simulink model "atrias_boom_nmStand_fullCtrl"  (R2015a)
settings: Solver=ode23t  StartTime=0.0  StopTime=t_end  FixedStep=0.001  MaxStep=1e-3  RelTol=1e-3
InitFcn:
  | addpath('../common/')
  | colors
StartFcn:
  | tic
StopFcn:
  | %stopscript
values from neighbouring files (symbols this model uses):
  A1_notch_f1 = -2*cos(fnotch_f1*sample_time)    [set_control_params.m]
  A2_notch_f1 = 1    [set_control_params.m]
  A_lpf_dtau = 1 + B1_lpf_dtau + B2_lpf_dtau    [set_control_params.m]
  ankle_stiffness = 1/2*pi    (= 1.57079632679)    [mechanical_params.m]
  B1_lpf_dtau = -2*exp(-lpf_damping*fcut_dtau*sample_time)*cos(fcut_dtau*sample_time*sqrt(1-lpf_damping^2))    [set_control_params.m]
  B1_notch_f1 = -2*exp(-notch_damping*fnotch_f1*sample_time)*cos(fnotch_f1*sample_time*sqrt(1-notch_damping^2))    [set_control_params.m]
  B2_lpf_dtau = exp(-2*lpf_damping*fcut_dtau*sample_time)    [set_control_params.m]
  B2_notch_f1 = exp(-2*notch_damping*fnotch_f1*sample_time)    [set_control_params.m]
  b_hmotor = 0    [mechanical_params.m]
  b_leg_spring = 0.075*sqrt(k_leg_spring*0.5*.25^2)    [mechanical_params.m]
  b_rotor = 0*60/(2*pi)*9.725e-5    (= 0)    [mechanical_params.m]
  boom_mount_to_center_diagonal = boom_mount_to_center / cos(pitch_mount_angle)    [mechanical_params.m]    (also in set_control_params.m)
  breakaway_friction = [25 25 25 25]    [mechanical_params.m]
  contactThr = 0.35    [set_control_params.m]
  coulomb_friction = [20 20 20 20]    [mechanical_params.m]
  d_com = (d_hip_com_to_torso_com*m_torso)/(m_torso + num_legs*m_hshaft)    [mechanical_params.m]
  delta_phi_max = 160*pi/180    (= 2.79252680319)    [mechanical_params.m]    (also in set_control_params.m)
  delta_phi_max_buffer = 20*pi/180    (= 0.349065850399)    [set_control_params.m]
  delta_phi_max_dropoff = 2*pi/180    (= 0.0349065850399)    [set_control_params.m]
  delta_phi_min = 25.5*pi/180    (= 0.445058959259)    [mechanical_params.m]    (also in set_control_params.m)
  friction_linear_zone = [0.5 0.5 0.5 0.5].*pi/180    [mechanical_params.m]
  g = 9.803    [mechanical_params.m]    (also in set_control_params.m = 9.81)
  gain_nodes_sea_torque = [0,65,350,700]    [set_control_params.m]
  HIP_MTR_MAX_CONT_TORQUE = HIP_MTR_MAX_CONT_CURRENT*HIP_MOTOR_CONSTANT*HIP_MTR_GEAR_RATIO    (= 86.0016)    [set_control_params.m]
  HIP_MTR_MAX_TORQUE = max_current_hip*Kt_hip*N_h    (= 629.28)    [mechanical_params.m]
  initial_boom_pitch = 0    [mechanical_params.m]
  initial_boom_roll = asin((initial_com_height + boom_mount_to_com + boom_mount_to_center*tan(pitch_mount_angle) - (base_12(2) + yshaft_12(2))) / (l_boom + boom_mount_to_center_diagonal))    [mechanical_params.m]
  initial_boom_yaw = 0    [mechanical_params.m]
  initial_hip_roll = 0*pi/180    (= 0)    [mechanical_params.m]
  initial_winch_angle = -12 * pi/180    (= -0.209439510239)    [mechanical_params.m]
  k_gn = m_total*g/0.01    (= 57041.421916)    [mechanical_params.m]
  k_gt = m_total*g/0.1    (= 5704.1421916)    [mechanical_params.m]
  k_leg_spring = 4118.3    [mechanical_params.m]    (also in set_control_params.m)
  K_notch_f1 = (1+B1_notch_f1+B2_notch_f1)/(1+A1_notch_f1+A2_notch_f1)    [set_control_params.m]
  k_phi = 5000    [mechanical_params.m]
  k_sea = [4118.3 4118.3 4118.3 4118.3]    [set_control_params.m]
  Kb_leg = 0.121    [mechanical_params.m]
  kd_boom_roll_Ctrl = 0    [main_1_nmStand.m]    (also in main_2_nmStand_moveBoom.m)
  kd_lateral = 2*sqrt(kp_lateral*0.8)    [set_control_params.m]
  kd_shin_max = kd_pd_avoid_limits    (= 1000)    [set_control_params.m]
  kd_shin_min = kd_pd_avoid_limits    (= 1000)    [set_control_params.m]
  kd_splay_max = kd_pd_avoid_limits    (= 1000)    [set_control_params.m]
  kd_splay_min = kd_pd_avoid_limits    (= 1000)    [set_control_params.m]
  kd_thigh_max = kd_pd_avoid_limits    (= 1000)    [set_control_params.m]
  kd_thigh_min = kd_pd_avoid_limits    (= 1000)    [set_control_params.m]
  kd_winch = td_winch*kp_winch    (= 989.239577798)    [mechanical_params.m]
  kp_boom_roll_Ctrl = 0    [main_1_nmStand.m]    (also in main_2_nmStand_moveBoom.m)
  kp_lateral = 1000    [set_control_params.m]
  kp_sea_torque = [0.3, 0.3, 6.0, 6.0]    [set_control_params.m]
  kp_shin_max = kp_pd_avoid_limits    (= 5000)    [set_control_params.m]
  kp_shin_min = kp_pd_avoid_limits    (= 5000)    [set_control_params.m]
  kp_splay_max = kp_pd_avoid_limits    (= 5000)    [set_control_params.m]
  kp_splay_min = kp_pd_avoid_limits/10    (= 500)    [set_control_params.m]
  kp_thigh_max = kp_pd_avoid_limits    (= 5000)    [set_control_params.m]
  kp_thigh_min = kp_pd_avoid_limits    (= 5000)    [set_control_params.m]
  kp_winch = winch_gravity_comp/(3*pi/180)    (= 19784.791556)    [mechanical_params.m]
  Kt_leg = 0.121    [mechanical_params.m]
  l_boom = 1.8161    [mechanical_params.m]    (also in set_control_params.m)
  L_leg = 0.102e-3    (= 0.000102)    [mechanical_params.m]
  l_seg = 0.5    [mechanical_params.m]    (also in set_control_params.m)
  l_v = l_seg*cos(min_splay_angle/2)    [set_control_params.m]
  lateral_offset = 0.2    [set_control_params.m]
  lateral_target_angle_right = -6*pi/180    (= -0.10471975512)    [set_control_params.m]
  lateral_transition_force = 150    [set_control_params.m]
  LEG_MTR_MAX_TORQUE = max_current_leg * Kt_leg * N    (= 1210)    [mechanical_params.m]
  loaded_unloaded_torque_threshold = 65*ones(1,4)    [set_control_params.m]
  lowerleg_12 = 0.40    (= 0.4)    [mechanical_params.m]
  m_boom = 4.49    [mechanical_params.m]
  m_fblink = 0.46    [mechanical_params.m]    (also in set_control_params.m)
  m_foot = 0.0857    [mechanical_params.m]
  m_hshaft = 18    [mechanical_params.m]    (also in set_control_params.m = 20)
  m_leg = m_thigh + m_lowerleg + m_shin + m_fblink    (= 2.3438)    [mechanical_params.m]
  m_leg_motor = 18    [set_control_params.m]
  m_lowerleg = 0.4438    [mechanical_params.m]    (also in set_control_params.m)
  m_output_gear = 1e-5    (= 1e-05)    [mechanical_params.m]    (also in set_control_params.m)
  m_rotor = 1e-5    (= 1e-05)    [mechanical_params.m]    (also in set_control_params.m)
  m_shin = 0.75    [mechanical_params.m]    (also in set_control_params.m)
  m_thigh = 0.69    [mechanical_params.m]    (also in set_control_params.m)
  m_torso = 17.5    [mechanical_params.m]    (also in set_control_params.m = 17.9)
  m_total = num_legs*(m_hshaft + m_thigh + m_lowerleg + m_shin + m_fblink + 2*m_gearing) + m_torso    (= 58.18772)    [mechanical_params.m]    (also in set_control_params.m = 62.58772)
  m_virtual_gear = 1e-5    (= 1e-05)    [mechanical_params.m]    (also in set_control_params.m)
  m_yshaft = 12.89    [mechanical_params.m]
  max_current_leg = 200    [mechanical_params.m]
  max_sagittal_loaded_torque = 833    [set_control_params.m]
  max_sagittal_unloaded_torque = 267    [set_control_params.m]
  max_torque_lateral = min(MTR_HIP_MAX_CURRENT, HIP_CURRENT_LIMIT)*HIP_MOTOR_CONSTANT*HIP_MTR_GEAR_RATIO    [set_control_params.m]
  max_voltage_leg = 50    [mechanical_params.m]
  maximum_lateral_angle = 18*pi/180    (= 0.314159265359)    [set_control_params.m]
  min_splay_angle = 45*pi/180    (= 0.785398163397)    [set_control_params.m]
  min_splay_buffer = 1*pi/180    (= 0.0174532925199)    [set_control_params.m]
  min_splay_dropoff = 5*pi/180    (= 0.0872664625997)    [set_control_params.m]
  minimum_lateral_angle = -9.5*pi/180    (= -0.165806278939)    [set_control_params.m]
  mu_hmotor = 0.90    (= 0.9)    [mechanical_params.m]
  mu_motor = 0.85    [mechanical_params.m]
  mu_slide = 0.8    [mechanical_params.m]
  mu_stick = 0.9    [mechanical_params.m]
  N = 50    [mechanical_params.m]
  N_h = r_hip_shaft / r_hip_gearhead    (= 57)    [mechanical_params.m]
  phi_max_collision = -5*pi/180    (= -0.0872664625997)    [mechanical_params.m]
  phi_roll_max = pi + 16*pi/180    (= 3.42084533391)    [mechanical_params.m]
  phi_roll_min = pi - 9*pi/180    (= 2.98451302091)    [mechanical_params.m]
  phi_shin_max = 3*pi/2 + 17.5*pi/180    (= 5.01782159948)    [mechanical_params.m]    (also in set_control_params.m)
  phi_shin_max_buffer = 20*pi/180    (= 0.349065850399)    [set_control_params.m]
  phi_shin_max_dropoff = 2*pi/180    (= 0.0349065850399)    [set_control_params.m]
  phi_shin_min = pi - 45*pi/180    (= 2.35619449019)    [mechanical_params.m]    (also in set_control_params.m)
  phi_shin_min_buffer = 20*pi/180    (= 0.349065850399)    [set_control_params.m]
  phi_shin_min_dropoff = 2*pi/180    (= 0.0349065850399)    [set_control_params.m]
  phi_thigh_max = pi + 45*pi/180    (= 3.92699081699)    [mechanical_params.m]    (also in set_control_params.m)
  phi_thigh_max_buffer = 20*pi/180    (= 0.349065850399)    [set_control_params.m]
  phi_thigh_max_dropoff = 2*pi/180    (= 0.0349065850399)    [set_control_params.m]
  phi_thigh_min = pi/2 - 17.5*pi/180    (= 1.2653637077)    [mechanical_params.m]    (also in set_control_params.m)
  phi_thigh_min_buffer = 20*pi/180    (= 0.349065850399)    [set_control_params.m]
  phi_thigh_min_dropoff = 2*pi/180    (= 0.0349065850399)    [set_control_params.m]
  r_hip_gearhead = 0.009525    [mechanical_params.m]
  r_hip_shaft = 0.542925    [mechanical_params.m]
  R_leg = 0.052    [mechanical_params.m]
  r_rotor = 0.001    [mechanical_params.m]
  r_virtual_gear = N*r_rotor    (= 0.05)    [mechanical_params.m]
  releaseThr = 0.2    [set_control_params.m]
  sample_time = 0.001    [set_control_params.m]
  ... (+19 more)
undefined symbols (not defined in the file or in its folder): A_lpf_velocity, B1_lpf_velocity, B2_lpf_velocity, base_color_d, boom_color_d, c, c_jointstop, CtrlPar_theta0, eref, fblink_color_d, floor_color_d, FmaxBFSH, FmaxGLU, FmaxHAM, FmaxHFL, FmaxRF, FmaxVAS, foot_color_d, FPCtrlPar, hshaft_color_d, j_motor, K, lateral_motor_efficiency, LLCtrlPar, loptBFSH, loptGLU, loptHAM, loptHFL, loptRF, loptVAS, lowerleg_color_d, lslackBFSH, lslackGLU, lslackHAM, lslackHFL, lslackRF, lslackVAS, MidDelay_discrete, Newton, output_sample_time, phi12_max, phi12_min, phi23_max, phi23_min, phimaxRFk, phimaxVAS, phirefBFSH, phirefGLU, phirefHAMh, phirefHAMk, phirefHFL, phirefRFh, phirefRFk, phirefVAS, phiScaleRFk, phiScaleVAS, rad ... (+40)
libraries: sm_lib x210, nesl_utility x140, simulink x58, simulink_extras x26, fl_lib x16, mblibv1 x2, commnoisgen2 x1
(part 1 of 19)
settings Model: CovSFcnEnable=off  Creator=wmartin  LastModifiedBy=smsong
settings SolverCC: MaxOrder=2  MaxConsecutiveZCs=100  ZeroCrossAlgorithm=Adaptive  InsertRTBMode=Never (minimum delay)
settings DataIOCC: LimitDataPoints=off  SaveOutput=off  SignalLogging=off  DSMLogging=off  ReturnWorkspaceOutputs=on  OutputTimes=[0:1/30:45]
settings OptimizationCC: UseDivisionForNetSlopeComputation=UseDivisionForReciprocalsOfIntegersOnly  UseFloatMulNetSlope=on  EnhancedBackFolding=on  MemcpyThreshold=1024  EfficientFloat2IntCast=on  SimCompilerOptimization=on  AccelVerboseBuild=on
settings DebuggingCC: AlgebraicLoopMsg=none  UnconnectedInputMsg=none  UnconnectedOutputMsg=none  UnconnectedLineMsg=none  StateNameClashWarn=warning
settings ModelReferenceCC: UpdateModelReferenceTargets=IfOutOfDate
settings SFSimCC: SFSimOverflowDetection=off  SFSimEcho=off
settings RTWCC: BuildConfiguration=Faster Runs
settings GRTTargetCC: MatFileLogging=off  SupportNonFinite=off
settings ExplorerConfigSet: InternalSimMechanicsExplorerSettings="<ExplorerConfiguration><canonicalview>planar_xy</canonicalview><AnimationSetting><BasePlaybackSpeed>1.0</BasePlaybackSpeed><PlaybackSpeedFactor>0.125</PlaybackSpeedFactor></AnimationSetting><TilePanel><TileInfo><Tiles Columns=\"1\" Count=\"1\" Rows=\"1\"><Column Left=\"2\" Weight=\"1\"/><Column Left=\"1588\"/><Row Top=\"2\" Weight=\"1\"/><Row Top=\"952\"/><Tile Height=\"1\" Width=\"1\" X=\"0\" Y=\"0\"/></Tiles></TileInfo><SceneInfo><SceneViewer><BGColor><R>0.89803922176361084</R><G>0.89803922176361084</G><B>0.94901961088180542</B></BGColor><Camera><Position><X>-1.0172976619760759</X><Y>1.3199969515095897</Y><Z>-22.747176205923715</Z></Position><Center><X>-0.27726326662667389</X><Y>1.3791295214552792</Y><Z>-4.6807347637942138</Z></Center><Up><X>-0.0083020071872005</X><Y>0.9999612367266113</Y><Z>-0.0029328690475362912</Z></Up><Left>-2.242677151053444</Left><Right>2.242677151053444</Right><Bottom>-1.8717961855383056</Bottom><Top>1.8717961855383056</Top></Camera></SceneViewer></SceneInfo></TilePanel></ExplorerConfiguration>"

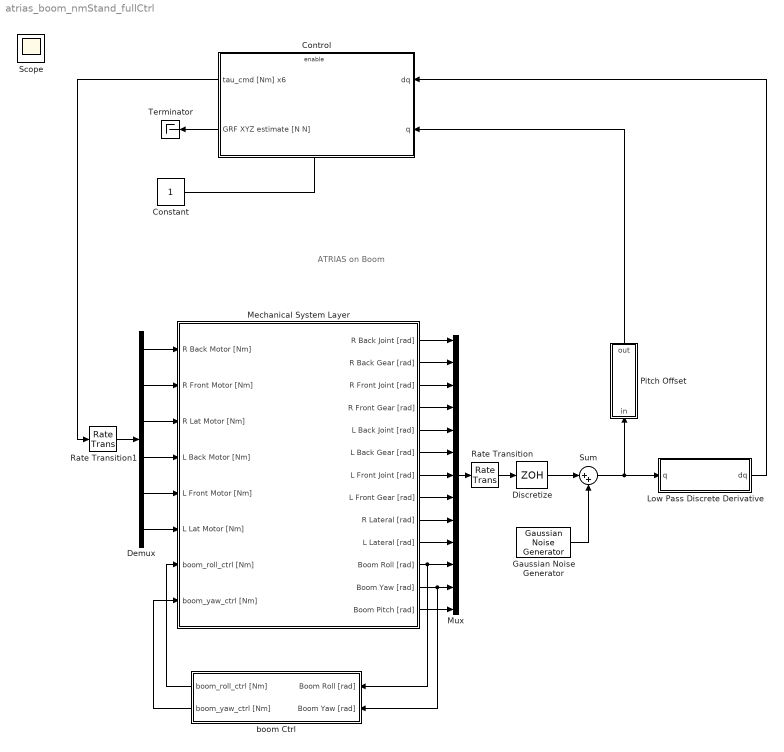
== system atrias_boom_nmStand_fullCtrl ==
  note: ATRIAS on Boom
  Constant : Constant
  Control : Subsystem
  Demux : Demux  Outputs=6
  Discretize : ZeroOrderHold  SampleTime=sample_time
  Gaussian Noise Generator : commnoisgen2/Gaussian Noise Generator  m=0  d=sensor_noise_variance  s=41  Ts=sample_time  frameBased=off  sampPerFrame=1  orient=off  outDataType=double
  Low Pass Discrete Derivative : Subsystem
  Mechanical System Layer : Subsystem
  Mux : Mux  Inputs=13
  Pitch Offset : Subsystem
  Rate Transition : RateTransition  OutPortSampleTime=sample_time
  Rate Transition1 : RateTransition  OutPortSampleTime=sample_time
  Sum : Sum  Inputs=|++
  Terminator : Terminator
  boom Ctrl : Subsystem
  Scope : Scope
      settings: SaveName=ScopeData35
  wires:
  Mechanical System Layer/1(R Back Joint [rad]) -> Mux/1
  Mechanical System Layer/2(R Back Gear [rad]) -> Mux/2
  Mechanical System Layer/3(R Front Joint [rad]) -> Mux/3
  Mechanical System Layer/4(R Front Gear [rad]) -> Mux/4
  Mechanical System Layer/5(L Back Joint [rad]) -> Mux/5
  Mechanical System Layer/6(L Back Gear [rad]) -> Mux/6
  Mechanical System Layer/7(L Front Joint [rad]) -> Mux/7
  Mechanical System Layer/8(L Front Gear [rad]) -> Mux/8
  Mechanical System Layer/9(R Lateral [rad]) -> Mux/9
  Mechanical System Layer/10(L Lateral [rad]) -> Mux/10
  Mechanical System Layer/11(Boom Roll [rad]) -> boom Ctrl/1(Boom Roll [rad]), Mux/11
  Mechanical System Layer/12(Boom Yaw [rad]) -> boom Ctrl/2(Boom Yaw [rad]), Mux/12
  Mechanical System Layer/13(Boom Pitch [rad]) -> Mux/13
  Mux/1 -> Rate Transition/1
  Demux/1 -> Mechanical System Layer/1(R Back Motor [Nm])
  Demux/2 -> Mechanical System Layer/2(R Front Motor [Nm])
  Demux/3 -> Mechanical System Layer/3(R Lat Motor [Nm])
  Demux/4 -> Mechanical System Layer/4(L Back Motor [Nm])
  Demux/5 -> Mechanical System Layer/5(L Front Motor [Nm])
  Demux/6 -> Mechanical System Layer/6(L Lat Motor [Nm])
  Discretize/1 -> Sum/1
  Gaussian Noise Generator/1 -> Sum/2
  Sum/1 -> Low Pass Discrete Derivative/1(q), Pitch Offset/1(in)
  Rate Transition1/1 -> Demux/1
  Rate Transition/1 -> Discretize/1
  Low Pass Discrete Derivative/1(dq) -> Control/1(dq)
  Control/1(tau_cmd [Nm] x6) -> Rate Transition1/1
  Constant/1 -> Control/Enable
  Pitch Offset/1(out) -> Control/2(q)
  Control/2(GRF XYZ estimate [N N]) -> Terminator/1
  boom Ctrl/1(boom_roll_ctrl [Nm]) -> Mechanical System Layer/7(boom_roll_ctrl [Nm])
  boom Ctrl/2(boom_yaw_ctrl [Nm]) -> Mechanical System Layer/8(boom_yaw_ctrl [Nm])

== system atrias_boom_nmStand_fullCtrl/Control ==
  dq : Inport
  q : Inport  Port=2
  Enable : EnablePort  StatesWhenEnabling=reset  PropagateVarSize=During execution
  Actuator Control : Subsystem
  Behavior Control : Subsystem
  tau_cmd [Nm] x6 : Outport  InitialOutput=[0 0 0 0 0 0]
  GRF XYZ estimate [N N] : Outport  Port=2  InitialOutput=[0 0 0]
  wires:
  q/1 -> Actuator Control/4(q), Behavior Control/2(q [rad] x13)
  dq/1 -> Actuator Control/5(dq), Behavior Control/1(dq [rad/s] x13)
  Behavior Control/1(Motor Torque Command [Nm] x6) -> Actuator Control/1(Desired Torque [Nm] x6)
  Actuator Control/1(tau_cmd [Nm] x6) -> tau_cmd [Nm] x6/1
  Behavior Control/2(SEA Torque Velocity Command [Nm] x4) -> Actuator Control/2(Desired SEA Torque Velocity [Nm] x4)
  Behavior Control/3(Force / Position Control [1/0] x4) -> Actuator Control/3(Enable SEA Control [1/0] x4)
  Behavior Control/4(GRF XYZ estimates [N N N]) -> GRF XYZ estimate [N N]/1

== system atrias_boom_nmStand_fullCtrl/Low Pass Discrete Derivative ==
  q : Inport
  Gain1 : Gain  Gain=1/sample_time
  discrete difference : Subsystem
  two_pole_filter : DiscreteTransferFcn  Numerator=[A_lpf_velocity 0 0]  Denominator=[1 B1_lpf_velocity B2_lpf_velocity]  SampleTime=sample_time
  dq : Outport
  wires:
  q/1 -> discrete difference/1(in)
  two_pole_filter/1 -> dq/1
  Gain1/1 -> two_pole_filter/1
  discrete difference/1(out) -> Gain1/1

== system atrias_boom_nmStand_fullCtrl/Mechanical System Layer ==
  R Back Motor [Nm] : Inport
  R Front Motor [Nm] : Inport  Port=2
  R Lat Motor [Nm] : Inport  Port=3
  L Back Motor [Nm] : Inport  Port=4
  L Front Motor [Nm] : Inport  Port=5
  L Lat Motor [Nm] : Inport  Port=6
  boom_roll_ctrl [Nm] : Inport  Port=7
  boom_yaw_ctrl [Nm] : Inport  Port=8
  Boom : Subsystem
      mask Display: image('../images/boom.png');
  Boom Base : Subsystem
      mask Display: image('../images/boom_base.png');
  Floor : Subsystem
  Floor Frame : sm_lib/Frames and Transforms/Rigid Transform  TranslationMethod=Cartesian  TranslationLengthUnit=m  TranslationStandardAxis=+Z  TranslationStandardOffset=0  TranslationCartesianOffset=[0 -0.03 0]  TranslationROffset=0  TranslationROffsetUnits=m  TranslationZOffset=0  TranslationZOffsetUnits=m  TranslationThetaOffset=0  TranslationThetaOffsetUnits=deg  RotationMethod=AlignedAxes  RotationAngleUnits=deg  RotationStandardAxis=+Z  RotationAngle=0  RotationArbitraryAxis=[0 0 1]  FollAlignAxisA=+Z  BaseAlignAxisA=+Y  FollAlignAxisB=+X  BaseAlignAxisB=+X  RotationMatrix=[1 0 0; 0 1 0; 0 0 1]  BlockFunction=simmechanics.library.frames_transforms.rigid_transform
  Ground : Subsystem
  Ground Contact Models : Subsystem
  L Hip Shaft : Subsystem
      mask Display: image(flipdim(imread('../images/hipshaft.JPG'),2));
  L Leg : Subsystem
      mask Display: image('../images/leg.JPG');
  Left Foot : Subsystem
      mask Display: image('../images/foot.png');
  Left Hip Roll Joint : Subsystem
  Pitch Joint : Subsystem
  R Hip Shaft : Subsystem
      mask Display: image('../images/hipshaft.JPG');
  R Leg : Subsystem
      mask Display: image('../images/leg.JPG');
  Right Foot : Subsystem
      mask Display: image('../images/foot.png');
  Right Hip Roll Joint : Subsystem
  Torso : Subsystem
      mask Display: image('../images/torso.png');
  Winch : Subsystem
  Yaw Joint : Subsystem
  Yaw Shaft : Subsystem
      mask Display: image('../images/boom_yaw_shaft.png');
  R Back Joint [rad] : Outport
  R Back Gear [rad] : Outport  Port=2
  R Front Joint [rad] : Outport  Port=3
  R Front Gear [rad] : Outport  Port=4
  L Back Joint [rad] : Outport  Port=5
  L Back Gear [rad] : Outport  Port=6
  L Front Joint [rad] : Outport  Port=7
  L Front Gear [rad] : Outport  Port=8
  R Lateral [rad] : Outport  Port=9
  L Lateral [rad] : Outport  Port=10
  Boom Roll [rad] : Outport  Port=11
  Boom Yaw [rad] : Outport  Port=12
  Boom Pitch [rad] : Outport  Port=13
  tag scope: qYaw=global
  wires:
  L Leg/1(Shin Joint [rad]) -> L Back Joint [rad]/1
  R Back Motor [Nm]/1 -> R Leg/1(Shin Motor [Nm])
  L Back Motor [Nm]/1 -> L Leg/1(Shin Motor [Nm])
  Right Hip Roll Joint/1(Hip Roll [rad]) -> R Lateral [rad]/1
  L Leg/3(Thigh Joint [rad]) -> L Front Joint [rad]/1
  Winch/1(Boom Roll [rad]) -> Boom Roll [rad]/1
  Left Hip Roll Joint/1(Hip Roll [rad]) -> L Lateral [rad]/1
  L Leg/4(Thigh Gear [rad]) -> L Front Gear [rad]/1
  R Leg/1(Shin Joint [rad]) -> R Back Joint [rad]/1
  R Leg/2(Shin Gear [rad]) -> R Back Gear [rad]/1
  L Leg/2(Shin Gear [rad]) -> L Back Gear [rad]/1
  R Leg/4(Thigh Gear [rad]) -> R Front Gear [rad]/1
  L Front Motor [Nm]/1 -> L Leg/2("Thigh Motor [Nm]  ")
  R Lat Motor [Nm]/1 -> Right Hip Roll Joint/1(Hip Motor [Nm])
  R Front Motor [Nm]/1 -> R Leg/2("Thigh Motor [Nm]  ")
  L Lat Motor [Nm]/1 -> Left Hip Roll Joint/1(Hip Motor [Nm])
  R Leg/3(Thigh Joint [rad]) -> R Front Joint [rad]/1
  Pitch Joint/1(Pitch [rad]) -> Boom Pitch [rad]/1
  Yaw Joint/1(Yaw [rad]) -> [qYaw], Boom Yaw [rad]/1
  boom_roll_ctrl [Nm]/1 -> Winch/1(boom_roll_ctrl [Nm])
  boom_yaw_ctrl [Nm]/1 -> Yaw Joint/1(boom_yaw_ctrl [Nm])
  connections:
  Torso/LConn1 -- Left Hip Roll Joint/RConn1
  Right Hip Roll Joint/RConn1 -- R Hip Shaft/RConn1
  Winch/RConn2 -- Yaw Shaft/RConn1
  Left Hip Roll Joint/LConn1 -- L Hip Shaft/LConn1
  Right Foot/LConn1 -- R Leg/LConn1
  R Leg/RConn1 -- R Hip Shaft/LConn1
  Torso/LConn2 -- Right Hip Roll Joint/LConn1
  L Leg/LConn1 -- L Hip Shaft/RConn1
  Left Foot/LConn1 -- L Leg/RConn1
  Pitch Joint/LConn1 -- Torso/RConn1
  Floor Frame/RConn1 -- Floor/LConn1
  Floor Frame/LConn1 -- Ground/RConn1 -- Boom Base/LConn1
  Boom/LConn1 -- Winch/RConn1
  Yaw Shaft/LConn1 -- Yaw Joint/RConn1
  Yaw Joint/LConn1 -- Boom Base/RConn1
  Pitch Joint/RConn1 -- Boom/RConn1
  Left Foot/RConn1 -- Ground Contact Models/RConn1
  Left Foot/RConn2 -- Ground Contact Models/RConn2
  Right Foot/RConn1 -- Ground Contact Models/RConn3
  Right Foot/RConn2 -- Ground Contact Models/RConn4

== system atrias_boom_nmStand_fullCtrl/Pitch Offset ==
  in : Inport
  1 to 12 : Selector  InputPortWidth=13  Indices=[1 2 3 4 5 6 7 8 9 10 11 12]
  13 : Selector  InputPortWidth=13  Indices=[13]
  Constant2 : Constant  Value=torso_centerline_pitch_offset_angle
  Mux : Mux  Inputs=2
  Sum : Sum  Inputs=++|
  out : Outport
  wires:
  1 to 12/1 -> Mux/1
  Mux/1 -> out/1
  Constant2/1 -> Sum/1
  in/1 -> 13/1, 1 to 12/1
  Sum/1 -> Mux/2
  13/1 -> Sum/2

== system atrias_boom_nmStand_fullCtrl/boom Ctrl ==
  Boom Roll [rad] : Inport
  Boom Yaw [rad] : Inport  Port=2
  Constant1 : Constant  Value=initial_boom_roll
  Constant3 : Constant  Value=initial_boom_roll
  Derivative : Derivative
  Derivative1 : Derivative
  Desired Roll Velocity1 : Constant  Value=0
  Desired Roll Velocity2 : Constant  Value=0
  Gain1 : Gain  Gain=kd_boom_roll_Ctrl
  Gain2 : Gain  Gain=kp_boom_roll_Ctrl
  Gain3 : Gain  Gain=kd_boom_roll_Ctrl
  Gain4 : Gain  Gain=kp_boom_roll_Ctrl
  Sum{1,3..4,6} (4 alike) : Sum  Inputs=+-|
  Sum2 : Sum  Inputs=+|+
  Sum5 : Sum  Inputs=+|+
  boom_roll_ctrl [Nm] : Outport
  boom_yaw_ctrl [Nm] : Outport  Port=2
  wires:
  Sum4/1 -> Gain2/1
  Desired Roll Velocity1/1 -> Sum6/1
  Sum6/1 -> Gain1/1
  Gain2/1 -> Sum5/1
  Gain1/1 -> Sum5/2
  Constant3/1 -> Sum4/1
  Boom Roll [rad]/1 -> Derivative/1, Sum4/2
  Sum5/1 -> boom_roll_ctrl [Nm]/1
  Derivative/1 -> Sum6/2
  Sum1/1 -> Gain4/1
  Desired Roll Velocity2/1 -> Sum3/1
  Sum3/1 -> Gain3/1
  Gain4/1 -> Sum2/1
  Gain3/1 -> Sum2/2
  Constant1/1 -> Sum1/1
  Boom Yaw [rad]/1 -> Derivative1/1, Sum1/2
  Sum2/1 -> boom_yaw_ctrl [Nm]/1
  Derivative1/1 -> Sum3/2

== system atrias_boom_nmStand_fullCtrl/Control/Actuator Control ==
  note: Order:
      | backR
      | frontR
      | backL
      | frontL
  note: Motor Order:
      |
      | backR
      | frontR
      | latR
      | backL
      | frontL
      | latL
  Desired Torque [Nm] x6 : Inport  OutDataTypeStr=double  PortDimensions=6  SampleTime=sample_time
  Desired SEA Torque Velocity [Nm] x4 : Inport  Port=2  OutDataTypeStr=double  PortDimensions=4  SampleTime=sample_time
  Enable SEA Control [1/0] x4 : Inport  Port=3  OutDataTypeStr=boolean  PortDimensions=4  SampleTime=sample_time
  q : Inport  Port=4  OutDataTypeStr=double  PortDimensions=13  SampleTime=sample_time
  dq : Inport  Port=5  OutDataTypeStr=double  PortDimensions=13  SampleTime=sample_time
  Activate SEA Control : Subsystem
  Antiresonance Compensation : Subsystem
  Hip Motor Efficiency Compensation : Gain  Gain=1/lateral_motor_efficiency
  Leg Motor Efficiency Compensation : Gain  Gain=1/sagittal_motor_efficiency
  Mux{1..2,4..5} (4 alike) : Mux
  Mux3 : Mux  Inputs=2
  SEA Control Toggle : Subsystem
  SEA Controller (Torque) : Subsystem
  Selector12 : Selector  InputPortWidth=13  Indices=[5 6]
  Selector13 : Selector  InputPortWidth=13  Indices=[7 8]
  Selector15 : Selector  InputPortWidth=13  Indices=[1 2]
  Selector16 : Selector  InputPortWidth=13  Indices=[3 4]
  Selector{17..20,25..28} (8 alike) : Selector  InputPortWidth=2  Indices=[1]
  Selector2 : Selector  InputPortWidth=13  Indices=[5 6]
  Selector{21..24,29..32} (8 alike) : Selector  InputPortWidth=2  Indices=[2]
  Selector3 : Selector  InputPortWidth=6  Indices=[3 6]
  Selector33 : Selector  InputPortWidth=6  Indices=[1 2 4 5]
  Selector4 : Selector  InputPortWidth=13  Indices=[7 8]
  Selector6 : Selector  InputPortWidth=13  Indices=[1 2]
  Selector7 : Selector  InputPortWidth=13  Indices=[3 4]
  Selector8 : Selector  InputPortWidth=6  Indices=[1 2 5 3 4 6]
  Selector9 : Selector  InputPortWidth=6  Indices=[1 2 4 5]
  Terminator1 : Terminator
  Torque Limiter (outside) 1 : Saturate  UpperLimit=max_sagittal_unloaded_torque  LowerLimit=-max_sagittal_unloaded_torque
      settings: AttributesFormatString=Hi: %<UpperLimit>\nLo: %<LowerLimit>
  tau_desired_signals : Gain  Description=xPCTag(1)=tau_cmd_signal;
  tau_cmd [Nm] x6 : Outport  OutDataTypeStr=double  PortDimensions=6  SampleTime=0  InitialOutput=[0 0 0 0 0 0]
  wires:
  Selector3/1 -> Hip Motor Efficiency Compensation/1
  [dqFrontL] -> Selector32/1
  Selector29/1 -> Mux5/1
  Selector18/1 -> Mux1/2
  Selector19/1 -> Mux1/3
  Selector2/1 -> [qBackL]
  Selector15/1 -> [dqBackR]
  dq/1 -> Selector13/1, Selector15/1, Selector16/1, Selector12/1
  tau_desired_signals/1 -> Terminator1/1
  Selector7/1 -> [qFrontR]
  Torque Limiter (outside) 1/1 -> Activate SEA Control/3(Torque Signal [Nm] x4), SEA Control Toggle/3(tau_cmd)
  Desired Torque [Nm] x6/1 -> Selector33/1, Selector9/1, Selector3/1, tau_desired_signals/1
  Selector8/1 -> tau_cmd [Nm] x6/1
  Selector6/1 -> [qBackR]
  SEA Controller (Torque)/1(tau_cmd sagittal [Nm] x4) -> Activate SEA Control/1(SEA Control Signal [Nm] x4)
  SEA Controller (Torque)/2(tau_measured [Nm] x4) -> SEA Control Toggle/2(tau_measured)
  Activate SEA Control/1(Torque Command [Nm] x4) -> Leg Motor Efficiency Compensation/1
  q/1 -> Selector2/1, Selector7/1, Selector6/1, Selector4/1
  Selector16/1 -> [dqFrontR]
  Selector4/1 -> [qFrontL]
  Selector9/1 -> Antiresonance Compensation/1(Torque)
  [qBackL] -> Selector23/1
  Selector26/1 -> Mux4/2
  Selector30/1 -> Mux5/2
  Mux5/1 -> SEA Controller (Torque)/6(dphi_gear [rad/s] x4)
  Leg Motor Efficiency Compensation/1 -> Mux3/1
  Selector24/1 -> Mux2/4
  [qFrontR] -> Selector18/1
  [qFrontL] -> Selector20/1
  [qBackR] -> Selector21/1
  Antiresonance Compensation/1(Filtered Torque) -> Torque Limiter (outside) 1/1
  Selector13/1 -> [dqFrontL]
  Selector23/1 -> Mux2/3
  Mux1/1 -> SEA Controller (Torque)/1(phi_load [rad] x4)
  [dqFrontL] -> Selector28/1
  Desired SEA Torque Velocity [Nm] x4/1 -> SEA Controller (Torque)/4(dtau_des sagittal [Nm] x4)
  Selector25/1 -> Mux4/1
  Selector31/1 -> Mux5/3
  [dqBackL] -> Selector31/1
  Hip Motor Efficiency Compensation/1 -> Mux3/2
  Selector28/1 -> Mux4/4
  [qFrontL] -> Selector24/1
  Selector22/1 -> Mux2/2
  [dqFrontR] -> Selector30/1
  Selector32/1 -> Mux5/4
  Mux4/1 -> SEA Controller (Torque)/5(dphi_load [rad/s] x4)
  Mux3/1 -> Selector8/1
  [dqBackR] -> Selector29/1
  Selector27/1 -> Mux4/3
  [qFrontR] -> Selector22/1
  Selector21/1 -> Mux2/1
  [dqBackL] -> Selector27/1
  [dqBackR] -> Selector25/1
  Selector20/1 -> Mux1/4
  Selector17/1 -> Mux1/1
  [qBackR] -> Selector17/1
  [qBackL] -> Selector19/1
  Selector12/1 -> [dqBackL]
  Mux2/1 -> SEA Controller (Torque)/2(phi_gear [rad] x4)
  SEA Control Toggle/1(SEA Control on/off [1/0]) -> Activate SEA Control/2("SEA on/off [1/0] x4 ")
  Selector33/1 -> SEA Controller (Torque)/3(tau_des sagittal [Nm] x4)
  Enable SEA Control [1/0] x4/1 -> SEA Control Toggle/1(enable)
  [dqFrontR] -> Selector26/1

== system atrias_boom_nmStand_fullCtrl/Control/Behavior Control ==
  note: Robot-NMM Interface
  note: Inputs
  note: Neuromuscular Model
  note: Avoid Limits
  note: Lateral Motors
  dq [rad/s] x13 : Inport
  q [rad] x13 : Inport  Port=2
  Add Limit Avoidance PD Torques : Subsystem
  Constant : Constant  Value=[0 0 0]
  Constant1 : Constant  Value=[1,1,1,1]
  Constant2 : Constant  Value=SEA_swing_ctrl_on_off
  Constant3 : Constant  Value=zeros(4,1)
  Data Type Conversion : DataTypeConversion  OutDataTypeStr=boolean
  Data Type Conversion1 : DataTypeConversion  OutDataTypeStr=boolean
  Demux3 : Demux
  Gain : Gain  Gain=-1
  Gain1 : Gain  Gain=-1
  Import Control Parameters : Subsystem
  Lateral Motor Control : Subsystem
  Mux : Mux  Inputs=6
  Mux1 : Mux  Inputs=2
  Mux3 : Mux  Inputs=2
  Mux5 : Mux  Inputs=2
  Mux7 : Mux
  Robot-to-NMM Interface : Subsystem
  Switch : Switch  Criteria=u2 ~= 0
  Terminator : Terminator
  Virtual Neuromuscular Control : Subsystem  SystemSampleTime=sample_time
  Motor Torque Command [Nm] x6 : Outport  OutputWhenDisabled=reset  InitialOutput=[0 0 0 0 0 0]
  SEA Torque Velocity Command [Nm] x4 : Outport  Port=2  OutputWhenDisabled=reset  InitialOutput=[0 0 0 0 0 0]
  Force / Position Control [1/0] x4 : Outport  Port=3  OutputWhenDisabled=reset  InitialOutput=[0 0 0 0 0 0]
  GRF XYZ estimates [N N N] : Outport  Port=4  OutputWhenDisabled=reset  InitialOutput=[0 0 0 0 0 0]
  tag scope: LFootCnt=global, LLLoad=global, LLat_ctrl_trq=global, LLength=global, Lalpha=global, LdLength=global, Ldalpha=global, Ldgamma=global, Lgamma=global, Lphi12=global, Lphi23=global, Lshin_ctrl_trq=global, Lshin_ctrl_trq_NMM=global, LtauB=global, LtauF=global, Lthigh_ctrl_trq=global, Lthigh_ctrl_trq_NMM=global, RFootCnt=global, RLLoad=global, RLat_ctrl_trq=global, RLength=global, Ralpha=global, RdLength=global, Rdalpha=global, Rdgamma=global, Rgamma=global, Rphi12=global, Rphi23=global, Rshin_ctrl_trq=global, Rshin_ctrl_trq_NMM=global, RtauB=global, RtauF=global, Rthigh_ctrl_trq=global, Rthigh_ctrl_trq_NMM=global, dq=global, k_L=global, k_R=global, q=global
  wires:
  q [rad] x13/1 -> [q]
  dq [rad/s] x13/1 -> [dq]
  [q] -> Robot-to-NMM Interface/1(q_discrete [rad] x13)
  [dq] -> Robot-to-NMM Interface/2(dq_discrete [rad/2] x13)
  Robot-to-NMM Interface/6(L Leg Load [bw]) -> [LLLoad]
  Robot-to-NMM Interface/5(R Leg Load [bw]) -> [RLLoad]
  Robot-to-NMM Interface/10(L Alpha [rad]) -> [Lalpha]
  Robot-to-NMM Interface/9(R Alpha [rad]) -> [Ralpha]
  Robot-to-NMM Interface/14(L Leg Length [m]) -> [LLength]
  Robot-to-NMM Interface/13(R Leg Length [m]) -> [RLength]
  Robot-to-NMM Interface/7(R Contact [0/1]) -> [RFootCnt]
  Robot-to-NMM Interface/8(L Contact [0/1]) -> [LFootCnt]
  Robot-to-NMM Interface/4(L_tau_front_meas [Nm]) -> [LtauF]
  Robot-to-NMM Interface/3(L_tau_back_meas [Nm]) -> [LtauB]
  Robot-to-NMM Interface/2(R_tau_front_meas [Nm]) -> [RtauF]
  Robot-to-NMM Interface/1(R_tau_back_meas [Nm]) -> [RtauB]
  Robot-to-NMM Interface/17(R virtual knee angle [rad]) -> [Rphi12]
  Robot-to-NMM Interface/18(R virtual hip angle [rad]) -> [Rphi23]
  Robot-to-NMM Interface/19(L virtual knee angle [rad]) -> [Lphi12]
  Robot-to-NMM Interface/20(L virtual hip angle [rad]) -> [Lphi23]
  Robot-to-NMM Interface/22(L Jacobian Constant (k)) -> [k_L]
  Robot-to-NMM Interface/21(R Jacobian Constant (k)) -> [k_R]
  Robot-to-NMM Interface/11(R dAlpha [rad/s]) -> [Rdalpha]
  Robot-to-NMM Interface/12(L dAlpha [rad/s]) -> [Ldalpha]
  Robot-to-NMM Interface/23(Rgamma [rad]) -> [Rgamma]
  Robot-to-NMM Interface/24(Lgamma [rad]) -> [Lgamma]
  Robot-to-NMM Interface/25(Rdgamma [rad]) -> [Rdgamma]
  Robot-to-NMM Interface/26(Ldgamma [rad]) -> [Ldgamma]
  Robot-to-NMM Interface/15(R Leg Length Velocity [m/s]) -> [RdLength]
  Robot-to-NMM Interface/16(L Leg Length Velocity [m/s]) -> [LdLength]
  Virtual Neuromuscular Control/1(RtauB_des [Nm]) -> [Rshin_ctrl_trq_NMM]
  Virtual Neuromuscular Control/2(RtauF_des [Nm]) -> [Rthigh_ctrl_trq_NMM]
  Virtual Neuromuscular Control/3(LtauB_des [Nm]) -> [Lshin_ctrl_trq_NMM]
  Virtual Neuromuscular Control/4(LtauF_des [Nm]) -> [Lthigh_ctrl_trq_NMM]
  [Rshin_ctrl_trq_NMM] -> Mux7/1
  [Rthigh_ctrl_trq_NMM] -> Mux7/2
  [Lshin_ctrl_trq_NMM] -> Mux7/3
  [Lthigh_ctrl_trq_NMM] -> Mux7/4
  Demux3/4 -> [Lthigh_ctrl_trq]
  Demux3/3 -> [Lshin_ctrl_trq]
  Demux3/2 -> [Rthigh_ctrl_trq]
  Demux3/1 -> [Rshin_ctrl_trq]
  [Rshin_ctrl_trq] -> Mux/1
  [Rthigh_ctrl_trq] -> Mux/2
  [RLat_ctrl_trq] -> Mux/3
  [Lshin_ctrl_trq] -> Mux/4
  [Lthigh_ctrl_trq] -> Mux/5
  [LLat_ctrl_trq] -> Mux/6
  Mux/1 -> Add Limit Avoidance PD Torques/1(tau_des [Nm] x6)
  Lateral Motor Control/2(tau_lateral_L) -> [LLat_ctrl_trq]
  Lateral Motor Control/1(tau_lateral_R) -> [RLat_ctrl_trq]
  Mux5/1 -> Mux1/2
  Mux3/1 -> Mux1/1
  [RFootCnt] -> Mux3/2, Mux3/1
  [LFootCnt] -> Mux5/1, Mux5/2
  Mux1/1 -> Data Type Conversion/1
  Constant1/1 -> Data Type Conversion1/1
  Data Type Conversion1/1 -> Switch/1
  Data Type Conversion/1 -> Switch/3
  Constant2/1 -> Switch/2
  Switch/1 -> Force / Position Control [1/0] x4/1
  Constant/1 -> GRF XYZ estimates [N N N]/1
  Mux7/1 -> Terminator/1
  Constant3/1 -> Demux3/1
  Add Limit Avoidance PD Torques/1(tau_des w/PD [Nm] x6) -> Gain/1
  Add Limit Avoidance PD Torques/2(d/dt[tau_des w/PD] [Nm/s] x4) -> Gain1/1
  Gain1/1 -> SEA Torque Velocity Command [Nm] x4/1
  Gain/1 -> Motor Torque Command [Nm] x6/1

== system atrias_boom_nmStand_fullCtrl/Low Pass Discrete Derivative/discrete difference ==
  note: q Order:
      |
      | backJointR
      | backGearR
      | frontJointR
      | frontGearR
      |
      | backJointL
      | backGearL
      | frontJointL
      | frontGearL
      |
      | latR
      | latL
      |
      | boomRoll
      | boomYaw
      | boomPitch
  in : Inport
  Demux : Demux  Outputs=13
  Mux : Mux  Inputs=13
  difference : simulink/Discrete/Difference  ICPrevInput=shin_initial_r  InputProcessing=Columns as channels (frame based)  OutMin=[]  OutMax=[]  OutDataType=fixdt(1, 16)  OutScaling=2^-10  DoSatur=off
  difference1 : simulink/Discrete/Difference  ICPrevInput=shin_initial_r  InputProcessing=Columns as channels (frame based)  OutMin=[]  OutMax=[]  OutDataType=fixdt(1, 16)  OutScaling=2^-10  DoSatur=off
  difference10 : simulink/Discrete/Difference  ICPrevInput=initial_boom_roll  InputProcessing=Columns as channels (frame based)  OutMin=[]  OutMax=[]  OutDataType=fixdt(1, 16)  OutScaling=2^-10  DoSatur=off
  difference11 : simulink/Discrete/Difference  ICPrevInput=initial_boom_yaw  InputProcessing=Columns as channels (frame based)  OutMin=[]  OutMax=[]  OutDataType=fixdt(1, 16)  OutScaling=2^-10  DoSatur=off
  difference12 : simulink/Discrete/Difference  ICPrevInput=initial_boom_pitch  InputProcessing=Columns as channels (frame based)  OutMin=[]  OutMax=[]  OutDataType=fixdt(1, 16)  OutScaling=2^-10  DoSatur=off
  difference2 : simulink/Discrete/Difference  ICPrevInput=thigh_initial_r  InputProcessing=Columns as channels (frame based)  OutMin=[]  OutMax=[]  OutDataType=fixdt(1, 16)  OutScaling=2^-10  DoSatur=off
  difference3 : simulink/Discrete/Difference  ICPrevInput=thigh_initial_r  InputProcessing=Columns as channels (frame based)  OutMin=[]  OutMax=[]  OutDataType=fixdt(1, 16)  OutScaling=2^-10  DoSatur=off
  difference4 : simulink/Discrete/Difference  ICPrevInput=shin_initial_l  InputProcessing=Columns as channels (frame based)  OutMin=[]  OutMax=[]  OutDataType=fixdt(1, 16)  OutScaling=2^-10  DoSatur=off
  difference5 : simulink/Discrete/Difference  ICPrevInput=shin_initial_l  InputProcessing=Columns as channels (frame based)  OutMin=[]  OutMax=[]  OutDataType=fixdt(1, 16)  OutScaling=2^-10  DoSatur=off
  difference6 : simulink/Discrete/Difference  ICPrevInput=thigh_initial_l  InputProcessing=Columns as channels (frame based)  OutMin=[]  OutMax=[]  OutDataType=fixdt(1, 16)  OutScaling=2^-10  DoSatur=off
  difference7 : simulink/Discrete/Difference  ICPrevInput=thigh_initial_l  InputProcessing=Columns as channels (frame based)  OutMin=[]  OutMax=[]  OutDataType=fixdt(1, 16)  OutScaling=2^-10  DoSatur=off
  difference8 : simulink/Discrete/Difference  ICPrevInput=initial_hip_roll  InputProcessing=Columns as channels (frame based)  OutMin=[]  OutMax=[]  OutDataType=fixdt(1, 16)  OutScaling=2^-10  DoSatur=off
  difference9 : simulink/Discrete/Difference  ICPrevInput=initial_hip_roll  InputProcessing=Columns as channels (frame based)  OutMin=[]  OutMax=[]  OutDataType=fixdt(1, 16)  OutScaling=2^-10  DoSatur=off
  out : Outport
  wires:
  Demux/1 -> difference/1
  in/1 -> Demux/1
  Mux/1 -> out/1
  Demux/2 -> difference1/1
  difference1/1 -> Mux/2
  Demux/3 -> difference2/1
  difference2/1 -> Mux/3
  Demux/4 -> difference3/1
  difference3/1 -> Mux/4
  Demux/5 -> difference4/1
  difference4/1 -> Mux/5
  Demux/6 -> difference5/1
  difference5/1 -> Mux/6
  Demux/7 -> difference6/1
  difference6/1 -> Mux/7
  Demux/8 -> difference7/1
  difference7/1 -> Mux/8
  Demux/9 -> difference8/1
  difference8/1 -> Mux/9
  Demux/10 -> difference9/1
  difference9/1 -> Mux/10
  Demux/11 -> difference10/1
  difference10/1 -> Mux/11
  Demux/12 -> difference11/1
  difference11/1 -> Mux/12
  Demux/13 -> difference12/1
  difference12/1 -> Mux/13
  difference/1 -> Mux/1

== system atrias_boom_nmStand_fullCtrl/Mechanical System Layer/Boom ==
  CS1 to CS2 : sm_lib/Frames and Transforms/Rigid Transform  TranslationMethod=Cartesian  TranslationLengthUnit=m  TranslationStandardAxis=+Z  TranslationStandardOffset=0  TranslationCartesianOffset=boom_12  TranslationROffset=0  TranslationROffsetUnits=m  TranslationZOffset=0  TranslationZOffsetUnits=m  TranslationThetaOffset=0  TranslationThetaOffsetUnits=deg  RotationMethod=None  RotationAngleUnits=deg  RotationStandardAxis=+Z  RotationAngle=0  RotationArbitraryAxis=[0 0 1]  FollAlignAxisA=+X  BaseAlignAxisA=+Y  FollAlignAxisB=+Y  BaseAlignAxisB=+Z  RotationMatrix=[1 0 0; 0 1 0; 0 0 1]  BlockFunction=simmechanics.library.frames_transforms.rigid_transform
  Frame Data : Subsystem
  Solid : sm_lib/Body Elements/Solid  InertiaType=Custom  Mass=m_boom  MassUnits=kg  CenterOfMass=com_boom  CenterOfMassUnits=m  MomentsOfInertia=i_boom_moments  MomentsOfInertiaUnits=kg*m^2  ProductsOfInertia=i_boom_products  ProductsOfInertiaUnits=kg*m^2  DensityBased=on  Density=1000  DensityUnits=kg/(m^3)  GraphicType=FromGeometry  MarkerShape=Sphere  MarkerSize=10  MarkerSizeUnits=m  GraphicVisPropType=AdvancedVisualProperties  GraphicDiffuseColor=boom_color_d  GraphicSpecularColor=[0.5 0.5 0.5 1.0]  GraphicAmbientColor=[boom_color_d*0.5 1.0]  GraphicEmissiveColor=[0.0 0.0 0.0 1.0]  GraphicShininess=128  GraphicOpacity=1.0  GeometryShape=FromFile  RectangleSize=[1 1]  RectangleSizeUnits=m  BrickDimensions=[1 1 1]  BrickDimensionUnits=m  CylinderRadius=l_rad  CylinderRadiusUnits=m  CylinderLength=l_seg  CylinderLengthUnits=m  SphereRadius=1  SphereRadiusUnits=m  EllipsoidRadii=[1 1 1]  EllipsoidRadiiUnits=m  ExtrusionCrossSection=[1 1; -1 1; -1 -1; 1 -1]  ExtrusionCrossSectionUnits=m  ExtrusionLength=1  ExtrusionLengthUnits=m  PolygonNumSides=3  PolygonOuterRadius=1  PolygonOuterRadiusUnits=m  ExtGeomFileType=STL  ExtGeomFileName=../models/boom_roll.stl  ExtGeomFileUnits=m  RevolutionCrossSection=[1 1; 1 -1; 2 -1; 2 1]  RevolutionCrossSectionUnits=m  RevolutionExtent=Full  RevolutionAngle=180  RevolutionAngleUnits=deg  BlockFunction=simmechanics.library.body_elements.solid
  CS1 : PMIOPort  Port=1  Side=Left
  CS2 : PMIOPort  Port=2  Side=Right
  connections:
  CS1/RConn1 -- Frame Data/LConn1 -- CS1 to CS2/LConn1 -- Solid/RConn1
  CS2/RConn1 -- CS1 to CS2/RConn1

== system atrias_boom_nmStand_fullCtrl/Mechanical System Layer/Boom Base ==
  CS1 to CS2 : sm_lib/Frames and Transforms/Rigid Transform  TranslationMethod=Cartesian  TranslationLengthUnit=m  TranslationStandardAxis=+Z  TranslationStandardOffset=0  TranslationCartesianOffset=base_12  TranslationROffset=0  TranslationROffsetUnits=m  TranslationZOffset=0  TranslationZOffsetUnits=m  TranslationThetaOffset=0  TranslationThetaOffsetUnits=deg  RotationMethod=None  RotationAngleUnits=deg  RotationStandardAxis=+Z  RotationAngle=0  RotationArbitraryAxis=[0 0 1]  FollAlignAxisA=+X  BaseAlignAxisA=+Y  FollAlignAxisB=+Y  BaseAlignAxisB=+Z  RotationMatrix=[1 0 0; 0 1 0; 0 0 1]  BlockFunction=simmechanics.library.frames_transforms.rigid_transform
  Solid : sm_lib/Body Elements/Solid  InertiaType=PointMass  Mass=0  MassUnits=kg  CenterOfMass=[0 0 0]  CenterOfMassUnits=m  MomentsOfInertia=[0 0 0]  MomentsOfInertiaUnits=kg*m^2  ProductsOfInertia=[0 0 0]  ProductsOfInertiaUnits=kg*m^2  DensityBased=on  Density=1000  DensityUnits=kg/(m^3)  GraphicType=FromGeometry  MarkerShape=Sphere  MarkerSize=10  MarkerSizeUnits=m  GraphicVisPropType=AdvancedVisualProperties  GraphicDiffuseColor=base_color_d  GraphicSpecularColor=[0.5 0.5 0.5 1.0]  GraphicAmbientColor=[base_color_d*0.5 1.0]  GraphicEmissiveColor=[0.0 0.0 0.0 1.0]  GraphicShininess=128  GraphicOpacity=1.0  GeometryShape=FromFile  RectangleSize=[1 1]  RectangleSizeUnits=m  BrickDimensions=[1 1 1]  BrickDimensionUnits=m  CylinderRadius=l_rad  CylinderRadiusUnits=m  CylinderLength=l_seg  CylinderLengthUnits=m  SphereRadius=1  SphereRadiusUnits=m  EllipsoidRadii=[1 1 1]  EllipsoidRadiiUnits=m  ExtrusionCrossSection=[1 1; -1 1; -1 -1; 1 -1]  ExtrusionCrossSectionUnits=m  ExtrusionLength=1  ExtrusionLengthUnits=m  PolygonNumSides=3  PolygonOuterRadius=1  PolygonOuterRadiusUnits=m  ExtGeomFileType=STL  ExtGeomFileName=../models/boom_base.stl  ExtGeomFileUnits=m  RevolutionCrossSection=[1 1; 1 -1; 2 -1; 2 1]  RevolutionCrossSectionUnits=m  RevolutionExtent=Full  RevolutionAngle=180  RevolutionAngleUnits=deg  BlockFunction=simmechanics.library.body_elements.solid
  CS1 : PMIOPort  Port=1  Side=Left
  CS2 : PMIOPort  Port=2  Side=Right
  connections:
  CS1 to CS2/LConn1 -- CS1/RConn1 -- Solid/RConn1
  CS2/RConn1 -- CS1 to CS2/RConn1
